simulink model "test_IDC"  (R2017a)
settings: Solver=VariableStepAuto  StartTime=0.0  StopTime=5  MaxStep=1e-5  RelTol=1e-3
libraries: slidercrank_basic_library_v1 x2
settings Model: Creator=filip  LastModifiedBy=filip

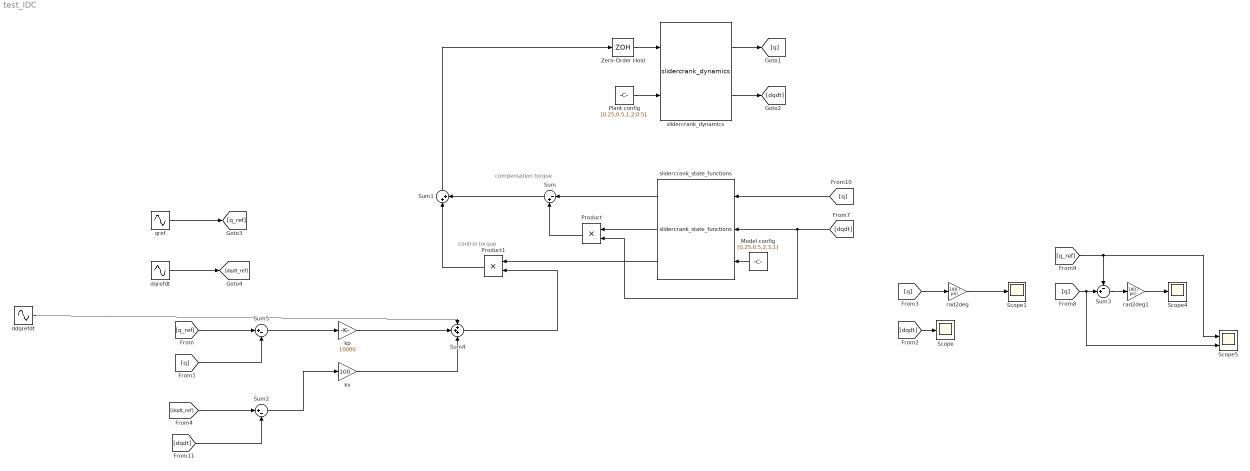
== system test_IDC ==
  note: compensation
      | torque
  note: control
      | torque
  Model config : Constant  Value=[0.25,0.5,2,3,1]
  Plant config : Constant  Value=[0.25,0.5,1,2,0.5]
  Product : Product
  Product1 : Product
  Scope : Scope
  Scope1 : Scope
  Scope4 : Scope
  Scope5 : Scope  NumInputPorts=2
  Sum : Sum  Inputs=|-+
  Sum1 : Sum  Inputs=|++
  Sum2 : Sum  Inputs=|+-
  Sum3 : Sum  Inputs=-+|
  Sum4 : Sum  Inputs=+++
  Sum5 : Sum  Inputs=|+-
  Zero-Order Hold : ZeroOrderHold  SampleTime=1e-3
  ddqrefdt : Sin  Amplitude=-100  Frequency=10  SampleTime=0
  dqrefdt : Sin  Amplitude=10  Frequency=10  Phase=pi()/2*10/2  SampleTime=0
  kp : Gain  Gain=10000
  kv : Gain  Gain=100
  qref : Sin  Frequency=10  SampleTime=0
  rad2deg : Gain  Gain=180 / pi()
  rad2deg1 : Gain  Gain=180 / pi()
  slidercrank_dynamics : slidercrank_basic_library_v1/slidercrank_dynamics
  slidercrank_state_functions : slidercrank_basic_library_v1/slidercrank_state_functions
  wires:
  Plant config/1 -> slidercrank_dynamics/2
  slidercrank_dynamics/1 -> [q]
  slidercrank_dynamics/2 -> [dqdt]
  [dqdt] -> Scope/1
  [q] -> rad2deg/1
  rad2deg/1 -> Scope1/1
  ddqrefdt/1 -> Sum4/1
  [q] -> Scope5/2, Sum3/2
  Sum3/1 -> rad2deg1/1
  rad2deg1/1 -> Scope4/1
  [q_ref] -> Scope5/1, Sum3/1
  Model config/1 -> slidercrank_state_functions/3
  [q] -> slidercrank_state_functions/1
  [dqdt] -> Product/2, slidercrank_state_functions/2
  slidercrank_state_functions/2 -> Product/1
  slidercrank_state_functions/1 -> Sum/1
  Product/1 -> Sum/2
  Sum/1 -> Sum1/2
  slidercrank_state_functions/3 -> Product1/1
  Product1/1 -> Sum1/1
  Sum4/1 -> Product1/2
  kp/1 -> Sum4/2
  kv/1 -> Sum4/3
  [dqdt_ref] -> Sum2/1
  [dqdt] -> Sum2/2
  Sum2/1 -> kv/1
  [q_ref] -> Sum5/1
  [q] -> Sum5/2
  Sum5/1 -> kp/1
  dqrefdt/1 -> [dqdt_ref]
  qref/1 -> [q_ref]
  Zero-Order Hold/1 -> slidercrank_dynamics/1
  Sum1/1 -> Zero-Order Hold/1
